simulink model "experiment3_matlab&simulink_practice"  (R2022a)
settings: Solver=VariableStepAuto  StartTime=0.0  StopTime=10  RelTol=1e-3
settings Model: Creator=slack  LastModifiedBy=slack

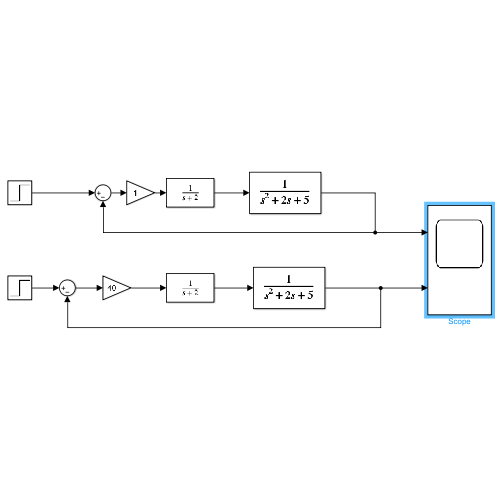
[thumbnail: Simulink's stored preview of the top-level diagram]
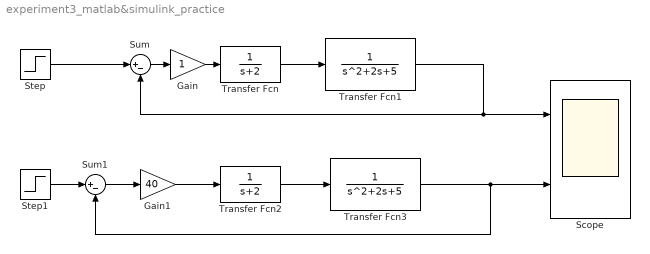
== system experiment3_matlab&simulink_practice ==
  Gain : Gain
  Gain1 : Gain  Gain=40
  Scope : Scope  NumInputPorts=2
  Step : Step  Time=0  After=20  SampleTime=0
  Step1 : Step  Time=0  SampleTime=0
  Sum : Sum  Inputs=|+-
  Sum1 : Sum  Inputs=|+-
  Transfer Fcn : TransferFcn  Denominator=[1 2]
  Transfer Fcn1 : TransferFcn  Denominator=[1 2 5]
  Transfer Fcn2 : TransferFcn  Denominator=[1 2]
  Transfer Fcn3 : TransferFcn  Denominator=[1 2 5]
  wires:
  Transfer Fcn/1 -> Transfer Fcn1/1
  Transfer Fcn1/1 -> Scope/1, Sum/2
  Transfer Fcn2/1 -> Transfer Fcn3/1
  Step/1 -> Sum/1
  Gain/1 -> Transfer Fcn/1
  Sum/1 -> Gain/1
  Transfer Fcn3/1 -> Sum1/2, Scope/2
  Sum1/1 -> Gain1/1
  Gain1/1 -> Transfer Fcn2/1
  Step1/1 -> Sum1/1
